simulink model "OutLoopInt_TestBed"  (R2012b)
settings: Solver=ode4  StartTime=0.0  StopTime=10  FixedStep=0.2  RelTol=1e-3
undefined symbols (not defined in the file): MWS
libraries: Lib_Solve_OuterLoopIntegrator_TMATS x1
settings Model: Creator=jwchapm2  LastModifiedBy=jwchapm2

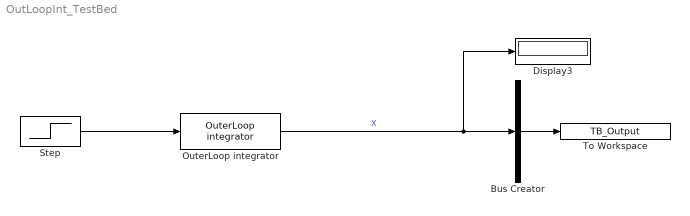
== system OutLoopInt_TestBed ==
  Bus Creator : BusCreator  Inputs=1
  Display3 : Display
  OuterLoop integrator : Lib_Solve_OuterLoopIntegrator_TMATS/OuterLoop integrator  OL_IC_M=MWS.OutLoopInt.IC
  Step : Step  Time=MWS.OutLoopInt.StepTime  Before=MWS.OutLoopInt.Inp1  After=MWS.OutLoopInt.Inp2  SampleTime=0
  To Workspace : ToWorkspace  VariableName=TB_Output  SampleTime=-1
  wires:
  Step/1 -> OuterLoop integrator/1
  OuterLoop integrator/1 -> Display3/1, Bus Creator/1  "X"
  Bus Creator/1 -> To Workspace/1
